simulink model "Assignment2_p7"  (R2020a)
settings: Solver=VariableStepAuto  StartTime=0.0  StopTime=100  RelTol=1e-3
libraries: simulink x1
settings Model: Creator=samrudh.untgodpr  LastModifiedBy=samrudh.untgodpr

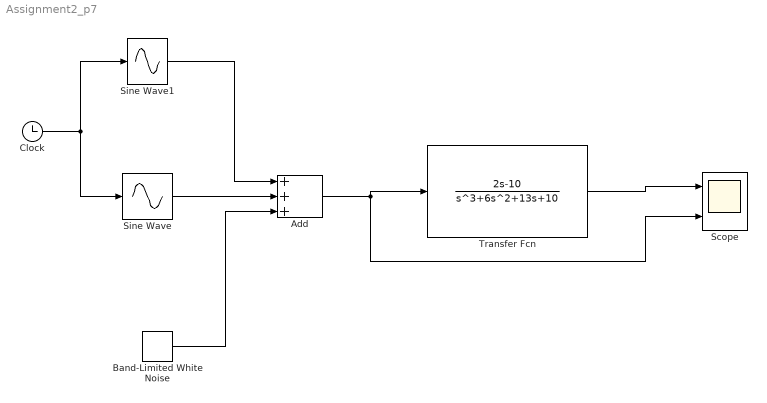
== system Assignment2_p7 ==
  Add : Sum  Inputs=+++
  Band-Limited White Noise : simulink/Sources/Band-Limited White Noise  Cov=[0.1]  Ts=100  seed=[23341]
  Clock : Clock
  Scope : Scope  NumInputPorts=2
  Sine Wave : Sin  TimeSource=Use external signal  Frequency=10  Phase=pi/3  SampleTime=0
  Sine Wave1 : Sin  TimeSource=Use external signal  Frequency=2  SampleTime=0
  Transfer Fcn : TransferFcn  Numerator=[2 -10]  Denominator=[1 6 13 10]
  wires:
  Sine Wave1/1 -> Add/1
  Sine Wave/1 -> Add/2
  Add/1 -> Transfer Fcn/1, Scope/2
  Transfer Fcn/1 -> Scope/1
  Band-Limited White Noise/1 -> Add/3
  Clock/1 -> Sine Wave/1, Sine Wave1/1
